simulink model "Modelling"  (R2020a)
settings: Solver=VariableStepAuto  StartTime=0.0  StopTime=10.0  RelTol=1e-3
PreLoadFcn:
  | ControllerToProject.m
values from neighbouring files (symbols this model uses):
  b = 8.2    [ControllerToProject.m]    (also in Parameters.m = 1)
  g = 9.81    [ControllerToProject.m]    (also in Parameters.m = 9.82)
  l = 0.36022    [ControllerToProject.m]    (also in Parameters.m = 0.35)
  mc = 0.9+0.1    (= 1)    [ControllerToProject.m]    (also in Parameters.m = 0.9)
  mp = 0.08887    [ControllerToProject.m]    (also in Parameters.m = 0.1)
undefined symbols (not defined in the file or in its folder): sigbuilder_block
libraries: simulink x4
settings Model: Creator=Emil  LastModifiedBy=Emil

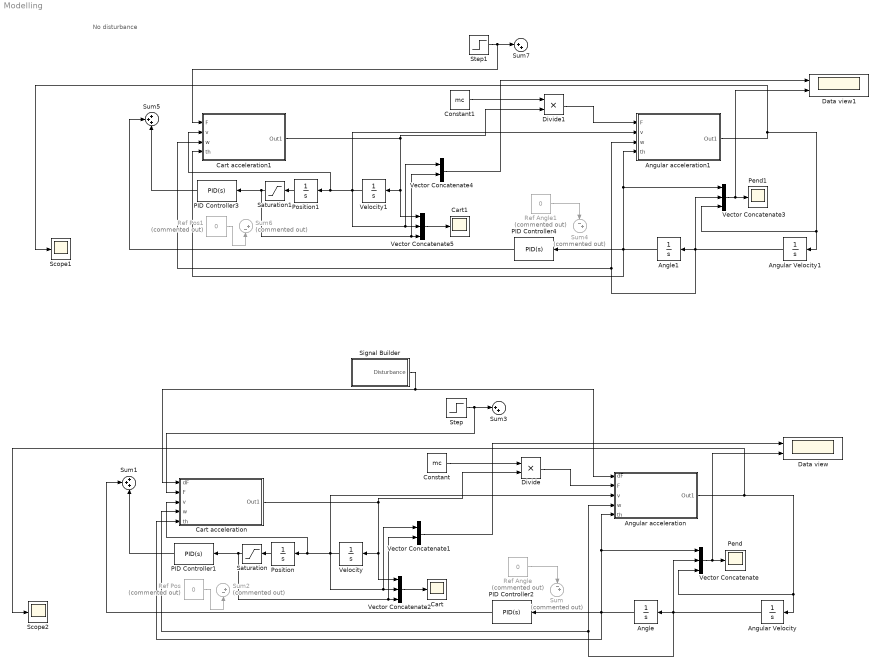
== system Modelling ==
  note: No disturbance
  Angle : Integrator
  Angle1 : Integrator
  Angular Velocity : Integrator
  Angular Velocity1 : Integrator
  Angular acceleration : Subsystem
  Angular acceleration1 : Subsystem
  Cart : Scope
  Cart acceleration : Subsystem
  Cart acceleration1 : Subsystem
  Cart1 : Scope
  Constant : Constant  Value=mc
  Constant1 : Constant  Value=mc
  Data view : Scope  NumInputPorts=2
  Data view1 : Scope  NumInputPorts=2
  Divide : Product  Inputs=**
  Divide1 : Product  Inputs=**
  PID Controller1 : simulink/Continuous/PID Controller  Controller=PID  Form=Ideal  TimeDomain=Continuous-time  UseExternalTs=off  SampleTime=-1  IntegratorMethod=Forward Euler  FilterMethod=Forward Euler  ControllerParametersSource=internal  P=-380.892958771882  I=0.42148790930739  D=0.173217560929601  UseFilter=on  N=5979.02668424825  TunerSelectOption=Transfer Function Based (PID Tuner App)  InitialConditionSource=internal  InitialConditionForIntegrator=0  InitialConditionForFilter=0  DifferentiatorICPrevScaledInput=0  ExternalReset=none  TrackingMode=off  Kt=1  LimitOutput=on  UpperSaturationLimit=5  LowerSaturationLimit=-5  LinearizeAsGain=on  AntiWindupMode=clamping  Kb=1  POutMin=[]  POutMax=[]  IOutMin=[]  IOutMax=[]  DOutMin=[]  DOutMax=[]  NOutMin=[]  NOutMax=[]  SumOutMin=[]  SumOutMax=[]  SaturationOutMin=[]  SaturationOutMax=[]  PParamMin=[]  PParamMax=[]  IParamMin=[]  IParamMax=[]  DParamMin=[]  DParamMax=[]  NParamMin=[]  NParamMax=[]  KbParamMin=[]  KbParamMax=[]  KtParamMin=[]  KtParamMax=[]  KbOutMin=[]  KbOutMax=[]  KtOutMin=[]  KtOutMax=[]  IntegratorOutMin=[]  IntegratorOutMax=[]  FilterOutMin=[]  FilterOutMax=[]  SumI1OutMin=[]  SumI1OutMax=[]  SumI2OutMin=[]  SumI2OutMax=[]  SumI3OutMin=[]  SumI3OutMax=[]  SumI4OutMin=[]  SumI4OutMax=[]  SumDOutMin=[]  SumDOutMax=[]  DifferentiatorOutMin=[]  DifferentiatorOutMax=[]  FilterDiffOutCoefMin=[]  FilterDiffOutCoefMax=[]  ReciprocalOutMin=[]  ReciprocalOutMax=[]  SumDenOutMin=[]  SumDenOutMax=[]  SumNumOutMin=[]  SumNumOutMax=[]  DivideOutMin=[]  DivideOutMax=[]  UdiffTsProdOutMin=[]  UdiffTsProdOutMax=[]  NTsProdOutMin=[]  NTsProdOutMax=[]  UintegralTsProdOutMin=[]  UintegralTsProdOutMax=[]  UngainTsProdOutMin=[]  UngainTsProdOutMax=[]  IntegratorContinuousStateAttributes=''  IntegratorStateMustResolveToSignalObject=off  IntegratorRTWStateStorageClass=Auto  FilterContinuousStateAttributes=''  FilterStateMustResolveToSignalObject=off  FilterRTWStateStorageClass=Auto  ParallelPVariant=Passthrough  IdealPVariant=InternalParameters  IVariant=InternalParameters  DVariant=InternalParameters  IntegratorVariant=Continuous  SatVariant=Enabled  AWVariant=ContClampingIdeal  PCopyVariant=InternalParamsIdeal  TRVariant=Disabled  FdbkBlocksVariant=Forward  IdealPFdbkVariant=Disabled  SatFdbkVariant=Disabled  DerivativeFilterVariant=ContFilter  NVariant=InternalParameters  NCopyVariant=Disabled  FilterICVariant=InternalICsFilter  IntegratorICVariant=InternalICs  ExternalResetVariant=Disabled  TRSumVariant=Passthrough  SumFdbkVariant=Disabled  SumVariant=Sum_PID  TsampFilterVariant=InternalTs  TsampNgainVariant=Passthrough  TsampIntegralVariant=Passthrough
  PID Controller2 : simulink/Continuous/PID Controller  Controller=PID  Form=Ideal  TimeDomain=Continuous-time  UseExternalTs=off  SampleTime=-1  IntegratorMethod=Forward Euler  FilterMethod=Forward Euler  ControllerParametersSource=internal  P=-1.40813056601747  I=7297.16708467672  D=0  UseFilter=on  N=100  TunerSelectOption=Transfer Function Based (PID Tuner App)  InitialConditionSource=internal  InitialConditionForIntegrator=0  InitialConditionForFilter=0  DifferentiatorICPrevScaledInput=0  ExternalReset=none  TrackingMode=off  Kt=1  LimitOutput=on  UpperSaturationLimit=5  LowerSaturationLimit=-5  LinearizeAsGain=on  AntiWindupMode=clamping  Kb=1  POutMin=[]  POutMax=[]  IOutMin=[]  IOutMax=[]  DOutMin=[]  DOutMax=[]  NOutMin=[]  NOutMax=[]  SumOutMin=[]  SumOutMax=[]  SaturationOutMin=[]  SaturationOutMax=[]  PParamMin=[]  PParamMax=[]  IParamMin=[]  IParamMax=[]  DParamMin=[]  DParamMax=[]  NParamMin=[]  NParamMax=[]  KbParamMin=[]  KbParamMax=[]  KtParamMin=[]  KtParamMax=[]  KbOutMin=[]  KbOutMax=[]  KtOutMin=[]  KtOutMax=[]  IntegratorOutMin=[]  IntegratorOutMax=[]  FilterOutMin=[]  FilterOutMax=[]  SumI1OutMin=[]  SumI1OutMax=[]  SumI2OutMin=[]  SumI2OutMax=[]  SumI3OutMin=[]  SumI3OutMax=[]  SumI4OutMin=[]  SumI4OutMax=[]  SumDOutMin=[]  SumDOutMax=[]  DifferentiatorOutMin=[]  DifferentiatorOutMax=[]  FilterDiffOutCoefMin=[]  FilterDiffOutCoefMax=[]  ReciprocalOutMin=[]  ReciprocalOutMax=[]  SumDenOutMin=[]  SumDenOutMax=[]  SumNumOutMin=[]  SumNumOutMax=[]  DivideOutMin=[]  DivideOutMax=[]  UdiffTsProdOutMin=[]  UdiffTsProdOutMax=[]  NTsProdOutMin=[]  NTsProdOutMax=[]  UintegralTsProdOutMin=[]  UintegralTsProdOutMax=[]  UngainTsProdOutMin=[]  UngainTsProdOutMax=[]  IntegratorContinuousStateAttributes=''  IntegratorStateMustResolveToSignalObject=off  IntegratorRTWStateStorageClass=Auto  FilterContinuousStateAttributes=''  FilterStateMustResolveToSignalObject=off  FilterRTWStateStorageClass=Auto  ParallelPVariant=Passthrough  IdealPVariant=InternalParameters  IVariant=InternalParameters  DVariant=InternalParameters  IntegratorVariant=Continuous  SatVariant=Enabled  AWVariant=ContClampingIdeal  PCopyVariant=InternalParamsIdeal  TRVariant=Disabled  FdbkBlocksVariant=Forward  IdealPFdbkVariant=Disabled  SatFdbkVariant=Disabled  DerivativeFilterVariant=ContFilter  NVariant=InternalParameters  NCopyVariant=Disabled  FilterICVariant=InternalICsFilter  IntegratorICVariant=InternalICs  ExternalResetVariant=Disabled  TRSumVariant=Passthrough  SumFdbkVariant=Disabled  SumVariant=Sum_PID  TsampFilterVariant=InternalTs  TsampNgainVariant=Passthrough  TsampIntegralVariant=Passthrough
  PID Controller3 : simulink/Continuous/PID Controller  Controller=PID  Form=Ideal  TimeDomain=Continuous-time  UseExternalTs=off  SampleTime=-1  IntegratorMethod=Forward Euler  FilterMethod=Forward Euler  ControllerParametersSource=internal  P=-380.892958771882  I=0.42148790930739  D=0.173217560929601  UseFilter=on  N=5979.02668424825  TunerSelectOption=Transfer Function Based (PID Tuner App)  InitialConditionSource=internal  InitialConditionForIntegrator=0  InitialConditionForFilter=0  DifferentiatorICPrevScaledInput=0  ExternalReset=none  TrackingMode=off  Kt=1  LimitOutput=on  UpperSaturationLimit=5  LowerSaturationLimit=-5  LinearizeAsGain=on  AntiWindupMode=clamping  Kb=1  POutMin=[]  POutMax=[]  IOutMin=[]  IOutMax=[]  DOutMin=[]  DOutMax=[]  NOutMin=[]  NOutMax=[]  SumOutMin=[]  SumOutMax=[]  SaturationOutMin=[]  SaturationOutMax=[]  PParamMin=[]  PParamMax=[]  IParamMin=[]  IParamMax=[]  DParamMin=[]  DParamMax=[]  NParamMin=[]  NParamMax=[]  KbParamMin=[]  KbParamMax=[]  KtParamMin=[]  KtParamMax=[]  KbOutMin=[]  KbOutMax=[]  KtOutMin=[]  KtOutMax=[]  IntegratorOutMin=[]  IntegratorOutMax=[]  FilterOutMin=[]  FilterOutMax=[]  SumI1OutMin=[]  SumI1OutMax=[]  SumI2OutMin=[]  SumI2OutMax=[]  SumI3OutMin=[]  SumI3OutMax=[]  SumI4OutMin=[]  SumI4OutMax=[]  SumDOutMin=[]  SumDOutMax=[]  DifferentiatorOutMin=[]  DifferentiatorOutMax=[]  FilterDiffOutCoefMin=[]  FilterDiffOutCoefMax=[]  ReciprocalOutMin=[]  ReciprocalOutMax=[]  SumDenOutMin=[]  SumDenOutMax=[]  SumNumOutMin=[]  SumNumOutMax=[]  DivideOutMin=[]  DivideOutMax=[]  UdiffTsProdOutMin=[]  UdiffTsProdOutMax=[]  NTsProdOutMin=[]  NTsProdOutMax=[]  UintegralTsProdOutMin=[]  UintegralTsProdOutMax=[]  UngainTsProdOutMin=[]  UngainTsProdOutMax=[]  IntegratorContinuousStateAttributes=''  IntegratorStateMustResolveToSignalObject=off  IntegratorRTWStateStorageClass=Auto  FilterContinuousStateAttributes=''  FilterStateMustResolveToSignalObject=off  FilterRTWStateStorageClass=Auto  ParallelPVariant=Passthrough  IdealPVariant=InternalParameters  IVariant=InternalParameters  DVariant=InternalParameters  IntegratorVariant=Continuous  SatVariant=Enabled  AWVariant=ContClampingIdeal  PCopyVariant=InternalParamsIdeal  TRVariant=Disabled  FdbkBlocksVariant=Forward  IdealPFdbkVariant=Disabled  SatFdbkVariant=Disabled  DerivativeFilterVariant=ContFilter  NVariant=InternalParameters  NCopyVariant=Disabled  FilterICVariant=InternalICsFilter  IntegratorICVariant=InternalICs  ExternalResetVariant=Disabled  TRSumVariant=Passthrough  SumFdbkVariant=Disabled  SumVariant=Sum_PID  TsampFilterVariant=InternalTs  TsampNgainVariant=Passthrough  TsampIntegralVariant=Passthrough
  PID Controller4 : simulink/Continuous/PID Controller  Controller=PID  Form=Ideal  TimeDomain=Continuous-time  UseExternalTs=off  SampleTime=-1  IntegratorMethod=Forward Euler  FilterMethod=Forward Euler  ControllerParametersSource=internal  P=-1.40813056601747  I=7297.16708467672  D=0  UseFilter=on  N=100  TunerSelectOption=Transfer Function Based (PID Tuner App)  InitialConditionSource=internal  InitialConditionForIntegrator=0  InitialConditionForFilter=0  DifferentiatorICPrevScaledInput=0  ExternalReset=none  TrackingMode=off  Kt=1  LimitOutput=on  UpperSaturationLimit=5  LowerSaturationLimit=-5  LinearizeAsGain=on  AntiWindupMode=clamping  Kb=1  POutMin=[]  POutMax=[]  IOutMin=[]  IOutMax=[]  DOutMin=[]  DOutMax=[]  NOutMin=[]  NOutMax=[]  SumOutMin=[]  SumOutMax=[]  SaturationOutMin=[]  SaturationOutMax=[]  PParamMin=[]  PParamMax=[]  IParamMin=[]  IParamMax=[]  DParamMin=[]  DParamMax=[]  NParamMin=[]  NParamMax=[]  KbParamMin=[]  KbParamMax=[]  KtParamMin=[]  KtParamMax=[]  KbOutMin=[]  KbOutMax=[]  KtOutMin=[]  KtOutMax=[]  IntegratorOutMin=[]  IntegratorOutMax=[]  FilterOutMin=[]  FilterOutMax=[]  SumI1OutMin=[]  SumI1OutMax=[]  SumI2OutMin=[]  SumI2OutMax=[]  SumI3OutMin=[]  SumI3OutMax=[]  SumI4OutMin=[]  SumI4OutMax=[]  SumDOutMin=[]  SumDOutMax=[]  DifferentiatorOutMin=[]  DifferentiatorOutMax=[]  FilterDiffOutCoefMin=[]  FilterDiffOutCoefMax=[]  ReciprocalOutMin=[]  ReciprocalOutMax=[]  SumDenOutMin=[]  SumDenOutMax=[]  SumNumOutMin=[]  SumNumOutMax=[]  DivideOutMin=[]  DivideOutMax=[]  UdiffTsProdOutMin=[]  UdiffTsProdOutMax=[]  NTsProdOutMin=[]  NTsProdOutMax=[]  UintegralTsProdOutMin=[]  UintegralTsProdOutMax=[]  UngainTsProdOutMin=[]  UngainTsProdOutMax=[]  IntegratorContinuousStateAttributes=''  IntegratorStateMustResolveToSignalObject=off  IntegratorRTWStateStorageClass=Auto  FilterContinuousStateAttributes=''  FilterStateMustResolveToSignalObject=off  FilterRTWStateStorageClass=Auto  ParallelPVariant=Passthrough  IdealPVariant=InternalParameters  IVariant=InternalParameters  DVariant=InternalParameters  IntegratorVariant=Continuous  SatVariant=Enabled  AWVariant=ContClampingIdeal  PCopyVariant=InternalParamsIdeal  TRVariant=Disabled  FdbkBlocksVariant=Forward  IdealPFdbkVariant=Disabled  SatFdbkVariant=Disabled  DerivativeFilterVariant=ContFilter  NVariant=InternalParameters  NCopyVariant=Disabled  FilterICVariant=InternalICsFilter  IntegratorICVariant=InternalICs  ExternalResetVariant=Disabled  TRSumVariant=Passthrough  SumFdbkVariant=Disabled  SumVariant=Sum_PID  TsampFilterVariant=InternalTs  TsampNgainVariant=Passthrough  TsampIntegralVariant=Passthrough
  Pend : Scope
  Pend1 : Scope
  Position : Integrator
  Position1 : Integrator
  Ref Angle : Constant  Commented=on  Value=0
  Ref Angle1 : Constant  Commented=on  Value=0
  Ref Pos : Constant  Commented=on  Value=0
  Ref Pos1 : Constant  Commented=on  Value=0
  Saturation : Saturate  UpperLimit=0.8  LowerLimit=-0.8
  Saturation1 : Saturate  UpperLimit=0.8  LowerLimit=-0.8
  Scope1 : Scope
  Scope2 : Scope
  Signal Builder : Subsystem  Tag=STV Subsys  LoadFcn=sigbuilder_block('load');  StartFcn=sigbuilder_block('start');  StopFcn=sigbuilder_block('stop');  ClipboardFcn=sigbuilder_block('clipboard');  mask(Sigbuilder block){tuvar=[0:10]}
      mask help: Simulink:masks:SigbuilderBlock_MD
      mask init:
      | if ~strcmp(get_param(bdroot(gcbh),'SimulationStatus'),'stopped') tuvar = sigbuilder_block('maskInit'); end
      settings: CopyFcn=sigbuilder_block('copy');  DeleteFcn=sigbuilder_block('delete');  ModelCloseFcn=sigbuilder_block('modelClose');  PreSaveFcn=sigbuilder_block('preSave');  PauseFcn=sigbuilder_block('pause');  ContinueFcn=sigbuilder_block('continue');  NameChangeFcn=sigbuilder_block('namechange');  OpenFcn=sigbuilder_block('open',[6 30 1428 681.75 ]);  CloseFcn=sigbuilder_block('close');
      mask Display: plot(0, 0, 100, 100,[2, 2, 32, 32, 2], [68, 8, 8, 68, 68],[32, 2], [38, 38], [32, 19, 2],[53, 60, 44], [32, 17, 17, 2],[16, 16, 31, 31]);txt = getActiveGroup(gcbh);text(2, 100, txt,'verticalAlignment', 'top');
  Step : Step  Before=1  After=0  SampleTime=0
  Step1 : Step  Before=1  After=0  SampleTime=0
  Sum : Sum  Commented=on  Inputs=-+|
  Sum1 : Sum  Inputs=+++
  Sum2 : Sum  Commented=on  Inputs=|+-
  Sum3 : Sum  Inputs=|++
  Sum4 : Sum  Commented=on  Inputs=-+|
  Sum5 : Sum  Inputs=+++
  Sum6 : Sum  Commented=on  Inputs=|+-
  Sum7 : Sum  Inputs=|++
  Vector Concatenate{,2..3,5} (4 alike) : Concatenate  NumInputs=3
  Vector Concatenate1 : Concatenate
  Vector Concatenate4 : Concatenate
  Velocity : Integrator
  Velocity1 : Integrator
  wires:
  Position/1 -> Saturation/1
  Velocity/1 -> Angular acceleration/3(v), Vector Concatenate2/2, Vector Concatenate1/1, Position/1, Cart acceleration/3(v)
  Cart acceleration/1(Out1) -> Divide/2, Velocity/1, Vector Concatenate2/1
  Angle/1 -> PID Controller2/1, Vector Concatenate/1, Angular acceleration/5(th), Cart acceleration/5(th)
  Angular acceleration/1(Out1) -> Scope2/1, Vector Concatenate/3, Angular Velocity/1
  Angular Velocity/1 -> Vector Concatenate/2, Angle/1, Cart acceleration/4(w), Angular acceleration/4(w)
  PID Controller1/1 -> Sum1/3
  PID Controller2/1 -> Sum1/2
  Constant/1 -> Divide/1
  Saturation/1 -> Vector Concatenate1/2, Vector Concatenate2/3, PID Controller1/1
  Ref Angle/1 -> Sum/1
  Ref Pos/1 -> Sum2/2
  Step/1 -> Cart acceleration/2(F), Sum3/1
  Vector Concatenate/1 -> Data view/2, Pend/1
  Vector Concatenate2/1 -> Cart/1
  Vector Concatenate1/1 -> Data view/1
  Divide/1 -> Angular acceleration/2(F)
  Signal Builder/1(Disturbance) -> Angular acceleration/1(dF), Cart acceleration/1(dF)
  PID Controller4/1 -> Sum5/2
  Position1/1 -> Saturation1/1
  Ref Pos1/1 -> Sum6/2
  Vector Concatenate3/1 -> Data view1/2, Pend1/1
  Step1/1 -> Cart acceleration1/1(F), Sum7/1
  Vector Concatenate4/1 -> Data view1/1
  Vector Concatenate5/1 -> Cart1/1
  Saturation1/1 -> Vector Concatenate4/2, Vector Concatenate5/3, PID Controller3/1
  Divide1/1 -> Angular acceleration1/1(F)
  Angular acceleration1/1(Out1) -> Scope1/1, Vector Concatenate3/3, Angular Velocity1/1
  PID Controller3/1 -> Sum5/3
  Angular Velocity1/1 -> Vector Concatenate3/2, Angle1/1, Cart acceleration1/3(w), Angular acceleration1/3(w)
  Constant1/1 -> Divide1/1
  Velocity1/1 -> Angular acceleration1/2(v), Vector Concatenate5/2, Vector Concatenate4/1, Position1/1, Cart acceleration1/2(v)
  Angle1/1 -> PID Controller4/1, Vector Concatenate3/1, Angular acceleration1/4(th), Cart acceleration1/4(th)
  Ref Angle1/1 -> Sum4/1
  Cart acceleration1/1(Out1) -> Divide1/2, Velocity1/1, Vector Concatenate5/1

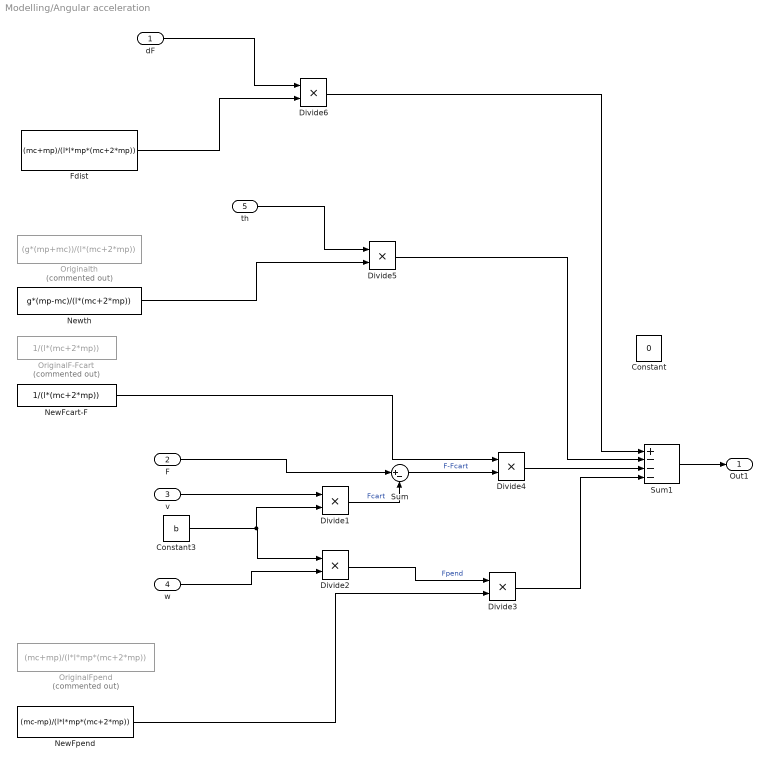
== system Modelling/Angular acceleration ==
  dF : Inport
  F : Inport  Port=2
  v : Inport  Port=3
  w : Inport  Port=4
  th : Inport  Port=5
  Constant : Constant  Value=0
  Constant3 : Constant  Value=b
  Divide{1..6} (6 alike) : Product  Inputs=**
  Fdist : Constant  Value=(mc+mp)/(l*l*mp*(mc+2*mp))
  NewFcart-F : Constant  Value=1/(l*(mc+2*mp))
  NewFpend : Constant  Value=(mc-mp)/(l*l*mp*(mc+2*mp))
  Newth : Constant  Value=g*(mp-mc)/(l*(mc+2*mp))
  OriginalF-Fcart : Constant  Commented=on  Value=1/(l*(mc+2*mp))
  OriginalFpend : Constant  Commented=on  Value=(mc+mp)/(l*l*mp*(mc+2*mp))
  Originalth : Constant  Commented=on  Value=(g*(mp+mc))/(l*(mc+2*mp))
  Sum : Sum  Inputs=|+-
  Sum1 : Sum  Inputs=+---
  Out1 : Outport
  wires:
  v/1 -> Divide1/1
  Constant3/1 -> Divide2/1, Divide1/2
  w/1 -> Divide2/2
  F/1 -> Sum/1
  Divide1/1 -> Sum/2  "Fcart"
  Divide2/1 -> Divide3/1  "Fpend"
  Sum/1 -> Divide4/2  "F-Fcart"
  th/1 -> Divide5/1
  Divide5/1 -> Sum1/2
  Divide4/1 -> Sum1/3
  Divide3/1 -> Sum1/4
  Sum1/1 -> Out1/1
  dF/1 -> Divide6/1
  Divide6/1 -> Sum1/1
  NewFpend/1 -> Divide3/2
  NewFcart-F/1 -> Divide4/1
  Newth/1 -> Divide5/2
  Fdist/1 -> Divide6/2

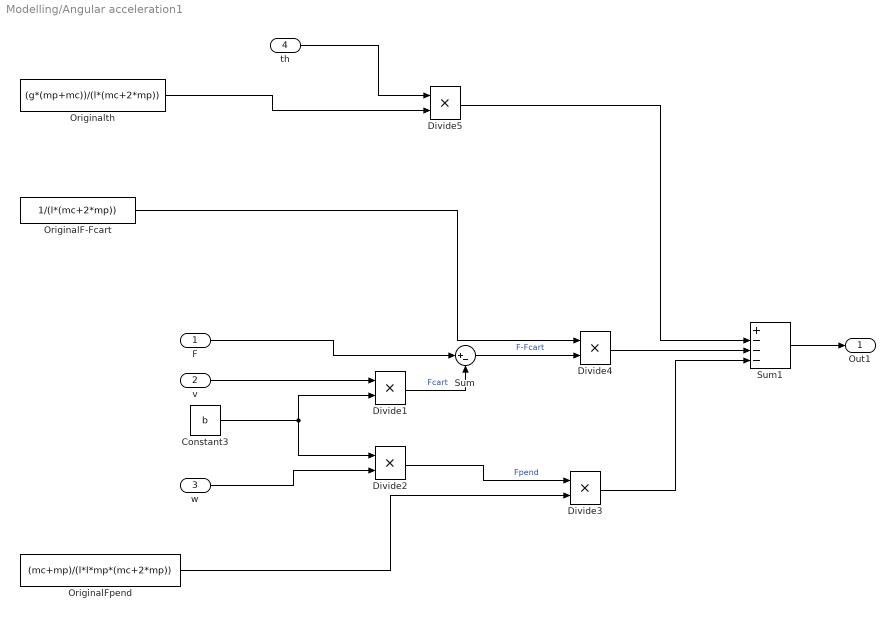
== system Modelling/Angular acceleration1 ==
  F : Inport
  v : Inport  Port=2
  w : Inport  Port=3
  th : Inport  Port=4
  Constant3 : Constant  Value=b
  Divide{1..5} (5 alike) : Product  Inputs=**
  OriginalF-Fcart : Constant  Value=1/(l*(mc+2*mp))
  OriginalFpend : Constant  Value=(mc+mp)/(l*l*mp*(mc+2*mp))
  Originalth : Constant  Value=(g*(mp+mc))/(l*(mc+2*mp))
  Sum : Sum  Inputs=|+-
  Sum1 : Sum  Inputs=+---
  Out1 : Outport
  wires:
  v/1 -> Divide1/1
  Constant3/1 -> Divide2/1, Divide1/2
  w/1 -> Divide2/2
  F/1 -> Sum/1
  Divide1/1 -> Sum/2  "Fcart"
  Divide2/1 -> Divide3/1  "Fpend"
  Sum/1 -> Divide4/2  "F-Fcart"
  th/1 -> Divide5/1
  Divide5/1 -> Sum1/2
  Divide4/1 -> Sum1/3
  Divide3/1 -> Sum1/4
  Sum1/1 -> Out1/1
  Originalth/1 -> Divide5/2
  OriginalF-Fcart/1 -> Divide4/1
  OriginalFpend/1 -> Divide3/2

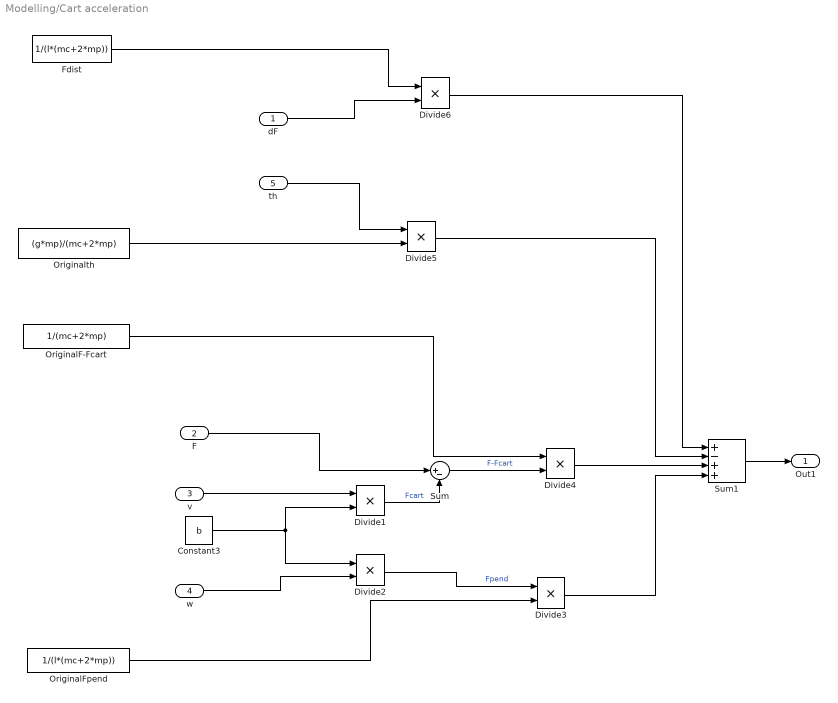
== system Modelling/Cart acceleration ==
  dF : Inport
  F : Inport  Port=2
  v : Inport  Port=3
  w : Inport  Port=4
  th : Inport  Port=5
  Constant3 : Constant  Value=b
  Divide{1..6} (6 alike) : Product  Inputs=**
  Fdist : Constant  Value=1/(l*(mc+2*mp))
  OriginalF-Fcart : Constant  Value=1/(mc+2*mp)
  OriginalFpend : Constant  Value=1/(l*(mc+2*mp))
  Originalth : Constant  Value=(g*mp)/(mc+2*mp)
  Sum : Sum  Inputs=|+-
  Sum1 : Sum  Inputs=+-++
  Out1 : Outport
  wires:
  v/1 -> Divide1/1
  Constant3/1 -> Divide2/1, Divide1/2
  w/1 -> Divide2/2
  F/1 -> Sum/1
  Divide1/1 -> Sum/2  "Fcart"
  Divide2/1 -> Divide3/1  "Fpend"
  Sum/1 -> Divide4/2  "F-Fcart"
  th/1 -> Divide5/1
  Divide5/1 -> Sum1/2
  Divide4/1 -> Sum1/3
  Divide3/1 -> Sum1/4
  Sum1/1 -> Out1/1
  dF/1 -> Divide6/2
  Fdist/1 -> Divide6/1
  OriginalFpend/1 -> Divide3/2
  OriginalF-Fcart/1 -> Divide4/1
  Originalth/1 -> Divide5/2
  Divide6/1 -> Sum1/1

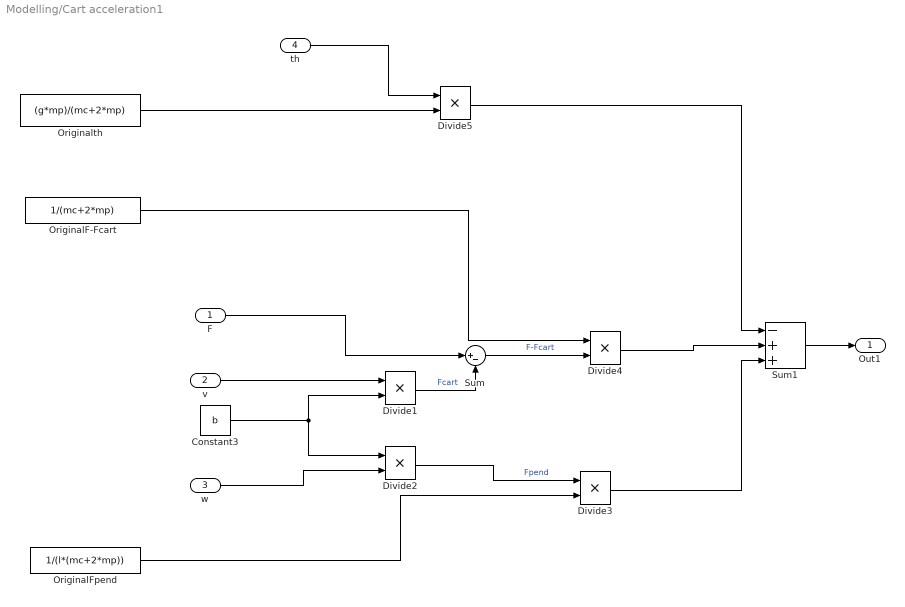
== system Modelling/Cart acceleration1 ==
  F : Inport
  v : Inport  Port=2
  w : Inport  Port=3
  th : Inport  Port=4
  Constant3 : Constant  Value=b
  Divide{1..5} (5 alike) : Product  Inputs=**
  OriginalF-Fcart : Constant  Value=1/(mc+2*mp)
  OriginalFpend : Constant  Value=1/(l*(mc+2*mp))
  Originalth : Constant  Value=(g*mp)/(mc+2*mp)
  Sum : Sum  Inputs=|+-
  Sum1 : Sum  Inputs=-++
  Out1 : Outport
  wires:
  v/1 -> Divide1/1
  Constant3/1 -> Divide2/1, Divide1/2
  w/1 -> Divide2/2
  F/1 -> Sum/1
  Divide1/1 -> Sum/2  "Fcart"
  Divide2/1 -> Divide3/1  "Fpend"
  Sum/1 -> Divide4/2  "F-Fcart"
  th/1 -> Divide5/1
  Divide5/1 -> Sum1/1
  Divide4/1 -> Sum1/2
  Divide3/1 -> Sum1/3
  Sum1/1 -> Out1/1
  OriginalFpend/1 -> Divide3/2
  OriginalF-Fcart/1 -> Divide4/1
  Originalth/1 -> Divide5/2

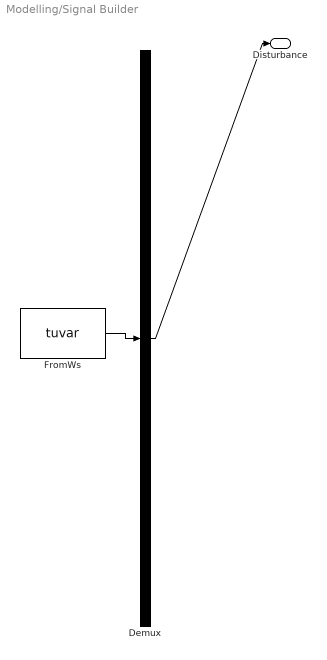
== system Modelling/Signal Builder ==
  Demux : Demux  Tag=STV Demux  Outputs=1
      settings: DisplayOption=none
  FromWs : FromWorkspace  Tag=STV FromWs  VariableName=tuvar
      SigBuilderData=|
      | common.afterFinalStr = 'Extrapolate'
      | common.sampleTime = 0
      | dataSet.timeRange = [0 10]
      | dataSet.name = 'Group 1'
      | sbobj.Groups.Name = 'Group 1'
      | sbobj.Groups.Signals.Name = 'Disturbance'
      | sbobj.Groups.Signals.XData = [0 0.25 0.5 0.75 1 1.25 1.5 1.75 2 2.25 2.5 2.75 3 3.25 3.5 3.75 4 4.25 4.5 4.75 5 5.25 5.5 5.75 6 6.25 6.5 6.75 7 7.25 7.5 7.75 8 8.25 8.5 8.75 9 9.25 9.5 9.75 10]
      | sbobj.Groups.Signals.YData = [0 0 0 0 0 0 0 0 0 0 0 -2.77555756156e-17 -0.002 0.063 0.002 -0.03 -0.05 -0.05 0.01 -0.146 0.16 0.08 0.1 0.089 0.193 0.06 0.02 -2.7756e-18 -0.022 -0.034 -0.099 -0.084 -0.01 -0.02 -0.051 -0.045 0.02 0.02 0.176 -2.7756e-18 -2.77555756156e-17]
  Disturbance : Outport  Tag=STV Outport
  wires:
  FromWs/1 -> Demux/1
  Demux/1 -> Disturbance/1
